simulink model "purePursuitBackward"  (R2024b)
settings: Solver=VariableStepAuto  StartTime=0.0  StopTime=4  RelTol=1e-3
PreLoadFcn:
  | setUpPurePursuitCurveLowVel
model workspace (MAT data in the model file):
  firstWarning = 0
  originalScenarioChecksum = 'F73A6DA3C723D3CA73A6F931B7A52A9C'
values from neighbouring files (symbols this model uses):
  L = 3    [setUpPurePursuit.m]    (also in setUpPurePursuitCurveLowVel.m)
  ld = 5    [setUpPurePursuit.m]    (also in setUpPurePursuitCurveLowVel.m)
  waypoints = data(:, 1:2)    [setUpPurePursuit.m]    (also in setUpPurePursuitCurveLowVel.m)
undefined symbols (not defined in the file or in its folder): psi_o, X_o, xRef, Y_o, yRef
libraries: simulink_extras x2, robotalgslib x2, vehdynlibviscommon x1, Solver_SF x1, autolibshared x1
settings Model: PacingRate=0.700000  Creator=valakshe  LastModifiedBy=kejin
settings SolverCC: AlgebraicLoopSolver=TrustRegion
settings DebuggingCC: UnconnectedInputMsg=warning  UnconnectedOutputMsg=warning  UnconnectedLineMsg=warning
settings ModelReferenceCC: EnableRefExpFcnMdlSchedulingChecks=on
settings RTWCC: GPUComputeCapability=3.5  DLArmComputeVersion=19.05

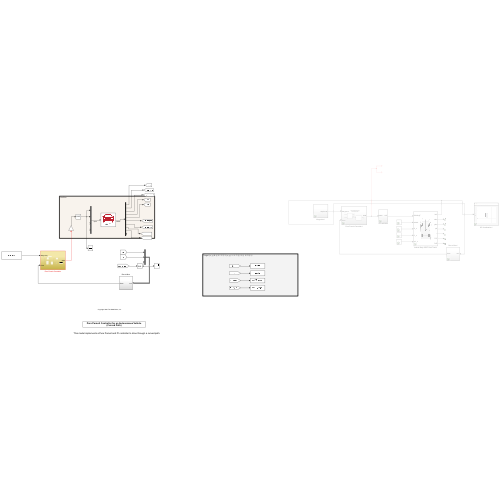
[thumbnail: Simulink's stored preview of the top-level diagram]
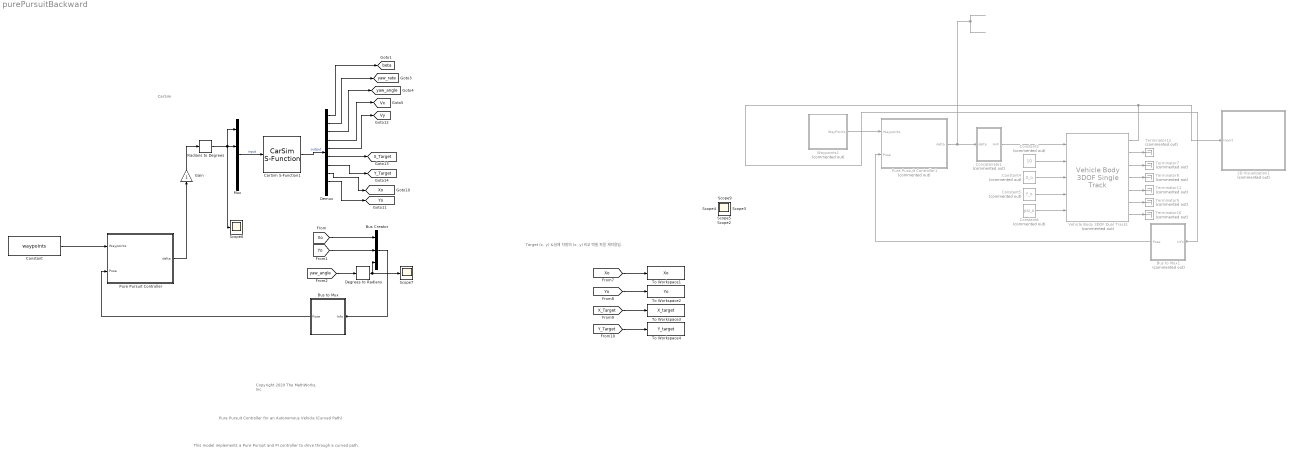
== system purePursuitBackward ==
  note: Copyright 2020 The MathWorks, Inc.
  note: Pure Pursuit Controller for an Autonomous Vehicle
      | (Curved Path)
  note: This model implements a Pure Pursuit and PI controller to drive through a curved path.
  note: CarSim
  note: Target (x, y) & 실제 차량의 (x, y) 비교 엑셀 파일 제작용임.
  2D Visualization1 : Subsystem  Commented=on
      mask Display: image("visualization.JPG");
  Bus Creator : BusCreator  Inputs=3
  Bus to Mux : Subsystem
  Bus to Mux1 : Subsystem  Commented=on
  CarSim S-Function1 : Solver_SF/CarSim S-Function  Priority=1  SIMFILE=simfile.sim  Run_RTs=off  vs_state_ind=Run  StopMode_ind=Vehicle Model
  Concatenate1 : Subsystem  Commented=on
  Constant : Constant  Value=waypoints
  Constant3 : Constant  Commented=on  Value=10
  Constant4 : Constant  Commented=on  Value=X_o
  Constant5 : Constant  Commented=on  Value=Y_o
  Constant6 : Constant  Commented=on  Value=psi_o
  Degrees to Radians : simulink_extras/Transformations/Degrees to Radians
  Demux : Demux  Outputs=10
  Gain : Gain
  Mux : Mux
  Pure Pursuit Controller : Subsystem
  Pure Pursuit Controller1 : Subsystem  Commented=on
  Radians to Degrees : simulink_extras/Transformations/Radians to Degrees
  Scope{,1..7,9} (9 alike) : Scope
  Terminator{7..12} (6 alike) : Terminator  Commented=on
  To Workspace1 : ToWorkspace  VariableName=Xo  SaveFormat=Timeseries  SampleTime=-1
  To Workspace2 : ToWorkspace  VariableName=Yo  SaveFormat=Timeseries  SampleTime=-1
  To Workspace3 : ToWorkspace  VariableName=X_target  SaveFormat=Timeseries  SampleTime=-1
  To Workspace4 : ToWorkspace  VariableName=Y_target  SaveFormat=Timeseries  SampleTime=-1
  Vehicle Body 3DOF Dual Track1 : autolibshared/Vehicle Body 3DOF Single Track  Commented=on  trackMode=Dual  inputMode=External longitudinal velocity  frontSteerMode=on  rearSteerMode=off  windMode=off  muMode=off  extFMode=off  extMMode=off  htchFMode=off  htchMMode=off  extXo=on  extpsio=on  extxdoto=off  extro=off  extYo=on  extTamb=off  extydoto=off  aMode=2  NF=2  NR=2  m=2000  a=1.4  b=1.6  h=0.35  dh=1  hh=0.2  X_o=0  xdot_o=0  CalphaMode=off  sigmaMode=on  d=0  hl=0  w=[1.4,1.4]  Cy_f=12e3  Cy_r=11e3  sigma_f=.1  sigma_r=.1  alpha_f_brk=[-.1 .1]  Cy_f_data=[-9e3 9e3]  alpha_r_brk=[-.1 .1]  Cy_r_data=[-9e3 9e3]  Y_o=0  ydot_o=0  Izz=4000  psi_o=0  r_o=0  Af=2  Cd=.3  Cl=.1  Cpm=.1  beta_w=[0:0.01:0.3]  Cs=[0:0.03:0.9]  Cym=[0:0.01:0.3]  Pabs=101325  Tair=273  g=9.81  mu=1  xdot_tol=.01  Fznom=5000  Fxtire_sat=7e4  Fytire_sat=7e4  longOff=0  latOff=0  vertOff=0  wrapAng=off
  Waypoints1 : Subsystem  Commented=on
  tag scope: Vx=global, Vy=global, X_Target=global, Xo=global, Y_Target=global, Yo=global, beta=global, yaw_angle=global, yaw_rate=global
  wires:
  Bus to Mux/1(Pose) -> Pure Pursuit Controller/2(Pose)
  Demux/3 -> [yaw_angle]
  Demux/6 -> [X_Target]
  Demux/7 -> [Y_Target]
  Demux/1 -> [beta]
  Demux/4 -> [Vx]
  Demux/5 -> [Vy]
  Mux/1 -> CarSim S-Function1/1  "input"
  CarSim S-Function1/1 -> Demux/1  "output"
  Demux/2 -> [yaw_rate]
  Demux/8 -> [Xo]
  Demux/9 -> [Yo]
  Vehicle Body 3DOF Dual Track1/5 -> Terminator11/1
  Bus to Mux1/1(Pose) -> Pure Pursuit Controller1/2(Pose)
  Vehicle Body 3DOF Dual Track1/4 -> Terminator8/1
  Vehicle Body 3DOF Dual Track1/2 -> Terminator12/1
  Constant4/1 -> Vehicle Body 3DOF Dual Track1/3
  Vehicle Body 3DOF Dual Track1/6 -> Terminator9/1
  Pure Pursuit Controller1/1(delta) -> Concatenate1/1(delta)
  Constant5/1 -> Vehicle Body 3DOF Dual Track1/4
  Constant6/1 -> Vehicle Body 3DOF Dual Track1/5
  Vehicle Body 3DOF Dual Track1/3 -> Terminator7/1
  Waypoints1/1(WayPoints) -> Pure Pursuit Controller1/1(Waypoints)
  Concatenate1/1(AnF) -> Vehicle Body 3DOF Dual Track1/1
  Vehicle Body 3DOF Dual Track1/7 -> Terminator10/1
  Vehicle Body 3DOF Dual Track1/1 -> Bus to Mux1/1(Info), 2D Visualization1/1(Inport)
  Constant3/1 -> Vehicle Body 3DOF Dual Track1/2
  Bus Creator/1 -> Bus to Mux/1(Info)
  [Xo] -> Bus Creator/1
  [Yo] -> Bus Creator/2
  [yaw_angle] -> Degrees to Radians/1
  [Y_Target] -> To Workspace4/1
  [Yo] -> To Workspace2/1
  [X_Target] -> To Workspace3/1
  [Xo] -> To Workspace1/1
  Degrees to Radians/1 -> Bus Creator/3, Scope7/1
  Radians to Degrees/1 -> Scope6/1, Mux/2, Mux/1
  Constant/1 -> Pure Pursuit Controller/1(Waypoints)
  Gain/1 -> Radians to Degrees/1
  Pure Pursuit Controller/1(delta) -> Gain/1

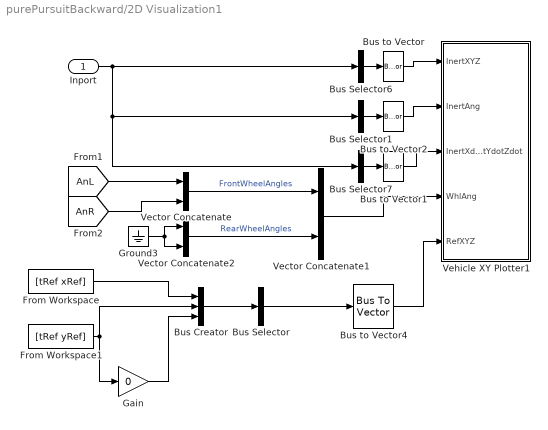
== system purePursuitBackward/2D Visualization1 ==
  Inport : Inport
  Bus Creator : BusCreator  Inputs=3
  Bus Selector : BusSelector  OutputSignals=signal1,signal2,signal3  OutputAsBus=on
  Bus Selector1 : BusSelector  OutputSignals=InertFrm.Cg.Ang.phi,InertFrm.Cg.Ang.theta,InertFrm.Cg.Ang.psi  OutputAsBus=on
  Bus Selector6 : BusSelector  OutputSignals=InertFrm.Geom.Disp.X,InertFrm.Geom.Disp.Y,InertFrm.Geom.Disp.Z  OutputAsBus=on
  Bus Selector7 : BusSelector  OutputSignals=InertFrm.Geom.Vel.Xdot,InertFrm.Geom.Vel.Ydot,InertFrm.Geom.Vel.Zdot  OutputAsBus=on
  Bus to Vector{,1..2,4} (4 alike) : BusToVector
  From Workspace : FromWorkspace  VariableName=[tRef xRef]
  From Workspace1 : FromWorkspace  VariableName=[tRef yRef]
  Gain : Gain  Gain=0
  Ground3 : Ground
  Vector Concatenate : Concatenate
  Vector Concatenate1 : Concatenate
  Vector Concatenate2 : Concatenate
  Vehicle XY Plotter1 : Subsystem  mask(Vehicle XY Plotter){extRef=on, extStats=off, extTireF=off, a=2, b=2, w=2, figBorder=10, bufferSize=1024, velNorm=5, tireFNorm=1000, pltDT=0.2}
      mask prompts: extRef "Plot path reference, extRef"; extStats "Display speed, RPM and Gear"; extTireF "Display tire forces"; a "Distance to front axle from CG, a [m]:"; b "Distance to rear axle from CG, b [m]:"; w "Track width, w [m]:"; figBorder "Distance to figure borders, figBorder [m]:"; bufferSize "Path buffer sampe size, bufferSize []:"; velNorm "Velocity vector scaling, velNorm [m*s/m]:"; tireFNorm "Tire force vector scaling, tireFNorm [m/N]:"; pltDT "Plot update rate, pltDT [s]:"
      mask help:
      | This block will display a MATLAB figure which indicates the vehicle path, current position and heading velocity.
      | An optional path reference is also provided.
      mask init:
      | block = gcb;
      | if autoblkschecksimstopped(block)
      |     ParamNames = {'extRef';'extStats';'extTireF';'extTireF'};
      |     PortNames = {'RefXYZ';'Stats';'TireFx';'TireFy'};
      |     for idx=1:length(PortNames)
      |         InportOption  = {'built-in/Ground', [PortNames{idx}, ' Ground'];...
      |             'built-in/Inport',PortNames{idx}};
      |         if ~strcmp(get_param(block,ParamNames{idx}),'on')
      |             NewBlkHdl = autoblksreplaceblock(block, InportOption, 1);
      |             set_param(NewBlkHdl, 'ShowName', 'off');
      |         else
      |             autoblksreplaceblock(block, InportOption, 2);
      |         end
      |     end
      |     InportNames = {'InertXYZ';'InertAng';'InertXdotYdotZdot';'WhlAng';'RefXYZ';'Stats';'TireFx';'TireFy'};
      |     FoundNames = get_param(find_system(block, 'LookUnderMasks', 'all', 'SearchDepth', 1, 'FollowLinks', 'on', 'BlockType', 'Inport'), 'Name');
      |     [~,PortI] = intersect(InportNames, FoundNames);
      |     PortI = sort(PortI);
      |     for idx = 1:length(PortI)
      |         set_param([block, '/', InportNames{PortI(idx)}], 'Port', num2str(idx));
      |     end
      | end
      mask TypeOptions a: Vehicle XY Plotter/a
      mask TypeOptions b: Vehicle XY Plotter/b
      mask TypeOptions w: Vehicle XY Plotter/w
      mask TypeOptions figBorder: Vehicle XY Plotter/figBorder
      mask TypeOptions bufferSize: Vehicle XY Plotter/bufferSize
      mask TypeOptions velNorm: Vehicle XY Plotter/velNorm
      mask TypeOptions tireFNorm: Vehicle XY Plotter/tireFNorm
      mask DialogControl Container3 Prompt: Plot and Display Options
  wires:
  Vector Concatenate1/1 -> Vehicle XY Plotter1/4(WhlAng)
  Ground3/1 -> Vector Concatenate2/1, Vector Concatenate2/2
  Bus Selector6/1 -> Bus to Vector/1
  Vector Concatenate/1 -> Vector Concatenate1/1  "FrontWheelAngles"
  [AnL] -> Vector Concatenate/1
  Vector Concatenate2/1 -> Vector Concatenate1/2  "RearWheelAngles"
  Bus Selector7/1 -> Bus to Vector1/1
  Bus to Vector1/1 -> Vehicle XY Plotter1/3(InertXdotYdotZdot)
  Bus to Vector/1 -> Vehicle XY Plotter1/1(InertXYZ)
  Bus to Vector2/1 -> Vehicle XY Plotter1/2(InertAng)
  Bus Selector1/1 -> Bus to Vector2/1
  [AnR] -> Vector Concatenate/2
  Inport/1 -> Bus Selector7/1, Bus Selector1/1, Bus Selector6/1
  Bus to Vector4/1 -> Vehicle XY Plotter1/5(RefXYZ)
  Bus Selector/1 -> Bus to Vector4/1
  From Workspace1/1 -> Gain/1, Bus Creator/2
  Gain/1 -> Bus Creator/3
  From Workspace/1 -> Bus Creator/1
  Bus Creator/1 -> Bus Selector/1

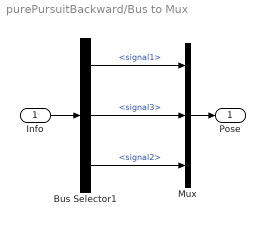
== system purePursuitBackward/Bus to Mux ==
  Info : Inport
  Bus Selector1 : BusSelector  OutputSignals=signal1,signal3,signal2
  Mux : Mux  Inputs=3
  Pose : Outport
  wires:
  Bus Selector1/3 -> Mux/3  "<signal2>"
  Bus Selector1/1 -> Mux/1  "<signal1>"
  Mux/1 -> Pose/1
  Bus Selector1/2 -> Mux/2  "<signal3>"
  Info/1 -> Bus Selector1/1

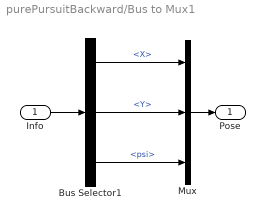
== system purePursuitBackward/Bus to Mux1 ==
  Info : Inport
  Bus Selector1 : BusSelector  OutputSignals=InertFrm.Cg.Disp.X,InertFrm.Cg.Disp.Y,InertFrm.Cg.Ang.psi
  Mux : Mux  Inputs=3
  Pose : Outport
  wires:
  Bus Selector1/3 -> Mux/3  "<psi>"
  Bus Selector1/1 -> Mux/1  "<X>"
  Mux/1 -> Pose/1
  Bus Selector1/2 -> Mux/2  "<Y>"
  Info/1 -> Bus Selector1/1

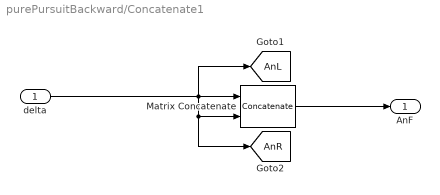
== system purePursuitBackward/Concatenate1 ==
  delta : Inport
  Matrix Concatenate : Concatenate
  AnF : Outport  VectorParamsAs1DForOutWhenUnconnected=off
  tag scope: AnL=global, AnR=global
  wires:
  Matrix Concatenate/1 -> AnF/1
  delta/1 -> [AnL], [AnR], Matrix Concatenate/2, Matrix Concatenate/1

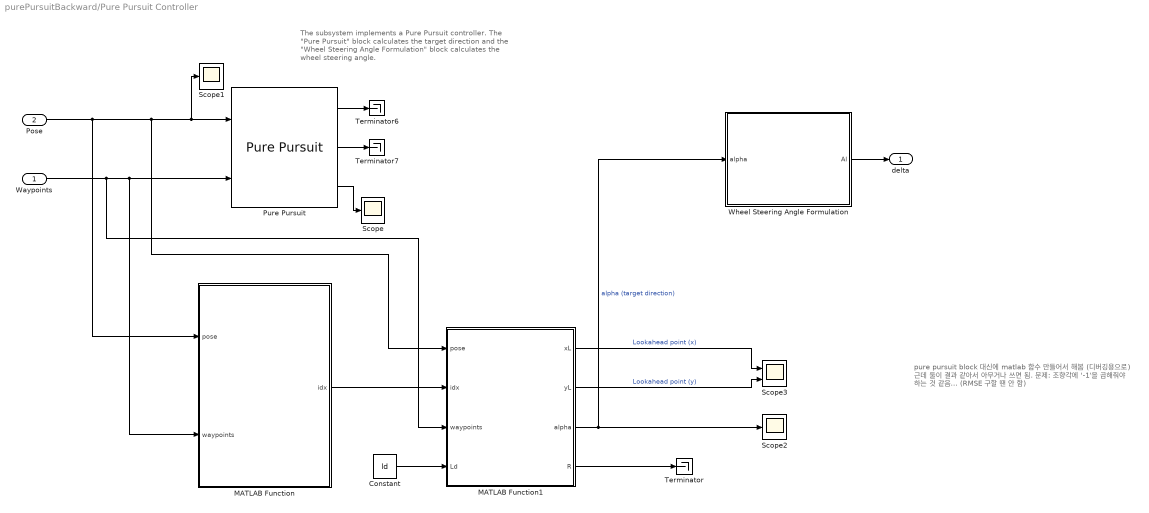
== system purePursuitBackward/Pure Pursuit Controller ==
  note: The subsystem implements a Pure Pursuit controller. The "Pure Pursuit" block calculates the target direction and the "Wheel Steering Angle Formulation" block calculates the wheel steering angle.
  note: pure pursuit block 대신에 matlab 함수 만들어서 해봄 (디버깅용으로)
      | 근데 둘이 결과 같아서 아무거나 쓰면 됨.
      | 문제: 조향각에 '-1'을 곱해줘야 하는 것 같음...
      | (RMSE 구할 땐 안 함)
  Waypoints : Inport
  Pose : Inport  Port=2
  Constant : Constant  Value=ld
  MATLAB Function : MATLAB Function  TreatAsAtomicUnit=on
  MATLAB Function1 : MATLAB Function  TreatAsAtomicUnit=on
  Pure Pursuit : robotalgslib/Pure Pursuit  DesiredLinearVelocityPort=off  DesiredLinearVelocity=0.1  MaxAngularVelocity=1.0  LookaheadDistancePort=off  LookaheadDistance=ld  TargetDirPort=on  SimulateUsing=Code generation
  Scope : Scope
  Scope1 : Scope
  Scope2 : Scope
  Scope3 : Scope  NumInputPorts=2
  Terminator : Terminator
  Terminator6 : Terminator
  Terminator7 : Terminator
  Wheel Steering Angle Formulation : Subsystem  mask{L=L, ld=ld}
      mask prompts: L "Bicycle length"; ld "Lookahead distance"
      mask TypeOptions L: Bicycle length/Value
      mask TypeOptions ld: Lookahead distance/Value
      mask Display:
      | image("GeometryMask.png")
      | port_label('input', 1, 'alpha')
      | port_label('output', 1, 'delta')
  delta : Outport
  wires:
  Wheel Steering Angle Formulation/1(Al) -> delta/1
  Pure Pursuit/3 -> Scope/1
  Waypoints/1 -> MATLAB Function1/3(waypoints), MATLAB Function/2(waypoints), Pure Pursuit/2
  Pure Pursuit/2 -> Terminator7/1
  Pose/1 -> MATLAB Function1/1(pose), Scope1/1, Pure Pursuit/1, MATLAB Function/1(pose)
  Pure Pursuit/1 -> Terminator6/1
  MATLAB Function/1(idx) -> MATLAB Function1/2(idx)
  Constant/1 -> MATLAB Function1/4(Ld)
  MATLAB Function1/3(alpha) -> Wheel Steering Angle Formulation/1(alpha), Scope2/1  "alpha (target direction)"
  MATLAB Function1/1(xL) -> Scope3/1  "Lookahead point (x)"
  MATLAB Function1/2(yL) -> Scope3/2  "Lookahead point (y)"
  MATLAB Function1/4(R) -> Terminator/1

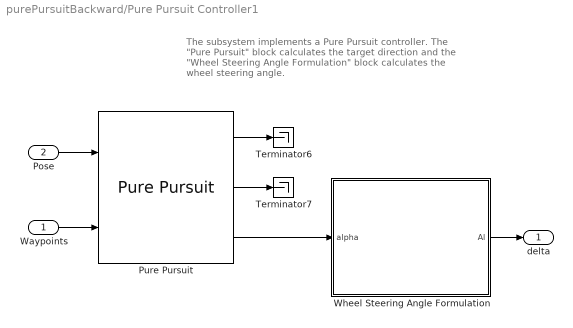
== system purePursuitBackward/Pure Pursuit Controller1 ==
  note: The subsystem implements a Pure Pursuit controller. The "Pure Pursuit" block calculates the target direction and the "Wheel Steering Angle Formulation" block calculates the wheel steering angle.
  Waypoints : Inport
  Pose : Inport  Port=2
  Pure Pursuit : robotalgslib/Pure Pursuit  DesiredLinearVelocityPort=off  DesiredLinearVelocity=0.1  MaxAngularVelocity=1.0  LookaheadDistancePort=off  LookaheadDistance=ld  TargetDirPort=on  SimulateUsing=Code generation
  Terminator6 : Terminator
  Terminator7 : Terminator
  Wheel Steering Angle Formulation : Subsystem  mask{L=L, ld=ld}
      mask prompts: L "Bicycle length"; ld "Lookahead distance"
      mask TypeOptions L: Bicycle length/Value
      mask TypeOptions ld: Lookahead distance/Value
      mask Display:
      | image("GeometryMask.png")
      | port_label('input', 1, 'alpha')
      | port_label('output', 1, 'delta')
  delta : Outport
  wires:
  Wheel Steering Angle Formulation/1(Al) -> delta/1
  Pure Pursuit/3 -> Wheel Steering Angle Formulation/1(alpha)
  Waypoints/1 -> Pure Pursuit/2
  Pure Pursuit/2 -> Terminator7/1
  Pose/1 -> Pure Pursuit/1
  Pure Pursuit/1 -> Terminator6/1

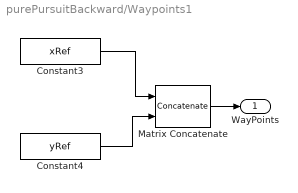
== system purePursuitBackward/Waypoints1 ==
  Constant3 : Constant  Value=xRef  SampleTime=0.1
  Constant4 : Constant  Value=yRef  SampleTime=0.1
  Matrix Concatenate : Concatenate  Mode=Multidimensional array  ConcatenateDimension=2
  WayPoints : Outport
  wires:
  Constant4/1 -> Matrix Concatenate/2
  Constant3/1 -> Matrix Concatenate/1
  Matrix Concatenate/1 -> WayPoints/1

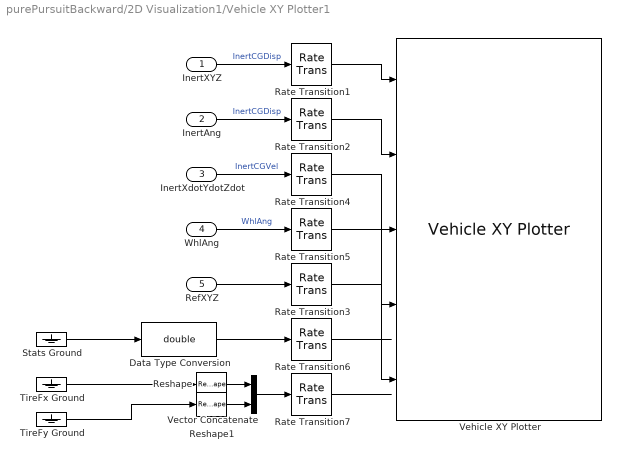
== system purePursuitBackward/2D Visualization1/Vehicle XY Plotter1 ==
  InertXYZ : Inport
  InertAng : Inport  Port=2
  InertXdotYdotZdot : Inport  Port=3
  WhlAng : Inport  Port=4
  RefXYZ : Inport  Port=5
  Data Type Conversion : DataTypeConversion  OutDataTypeStr=double  SaturateOnIntegerOverflow=off  RndMeth=Floor
  Rate Transition{1..7} (7 alike) : RateTransition  Deterministic=off  OutPortSampleTime=pltDT
  Reshape : Reshape  OutputDimensionality=Row vector (2-D)
  Reshape1 : Reshape  OutputDimensionality=Row vector (2-D)
  Stats Ground : Ground
  TireFx Ground : Ground
  TireFy Ground : Ground
  Vector Concatenate : Concatenate  Mode=Multidimensional array
  Vehicle XY Plotter : vehdynlibviscommon/Vehicle XY Plotter  w=w  a=a  b=b  figBorder=figBorder  bufferSize=bufferSize  extStats=off  extTireF=off
  wires:
  Vector Concatenate/1 -> Rate Transition7/1
  Reshape1/1 -> Vector Concatenate/2
  Reshape/1 -> Vector Concatenate/1
  RefXYZ/1 -> Rate Transition3/1
  Rate Transition7/1 -> ?
  Data Type Conversion/1 -> Rate Transition6/1
  Rate Transition6/1 -> ?
  Rate Transition5/1 -> Vehicle XY Plotter/4
  Rate Transition4/1 -> Vehicle XY Plotter/3
  Rate Transition2/1 -> Vehicle XY Plotter/2
  Rate Transition1/1 -> Vehicle XY Plotter/1
  Rate Transition3/1 -> Vehicle XY Plotter/5
  WhlAng/1 -> Rate Transition5/1  "WhlAng"
  InertXYZ/1 -> Rate Transition1/1  "InertCGDisp"
  InertXdotYdotZdot/1 -> Rate Transition4/1  "InertCGVel"
  InertAng/1 -> Rate Transition2/1  "InertCGDisp"
  TireFx Ground/1 -> Reshape/1
  TireFy Ground/1 -> Reshape1/1
  Stats Ground/1 -> Data Type Conversion/1

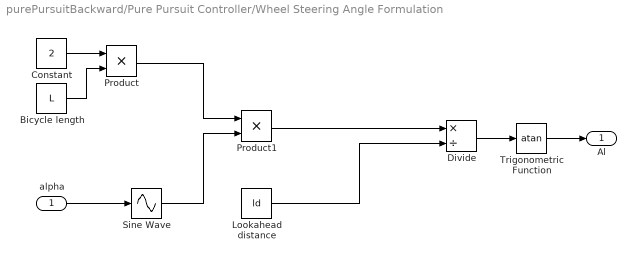
== system purePursuitBackward/Pure Pursuit Controller/Wheel Steering Angle Formulation ==
  alpha : Inport
  Bicycle length : Constant  Value=L
  Constant : Constant  Value=2
  Divide : Product  Inputs=*/
  Lookahead distance : Constant  Value=ld
  Product : Product
  Product1 : Product
  Sine Wave : Sin  TimeSource=Use external signal  SampleTime=0
  Trigonometric Function : Trigonometry  Operator=atan
  Al : Outport
  wires:
  Sine Wave/1 -> Product1/2
  Constant/1 -> Product/1
  Product1/1 -> Divide/1
  Product/1 -> Product1/1
  Divide/1 -> Trigonometric Function/1
  Trigonometric Function/1 -> Al/1
  alpha/1 -> Sine Wave/1
  Bicycle length/1 -> Product/2
  Lookahead distance/1 -> Divide/2

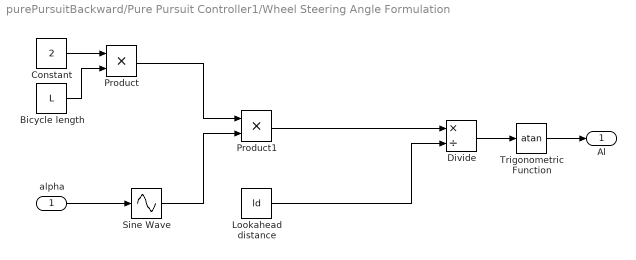
== system purePursuitBackward/Pure Pursuit Controller1/Wheel Steering Angle Formulation ==
  alpha : Inport
  Bicycle length : Constant  Value=L
  Constant : Constant  Value=2
  Divide : Product  Inputs=*/
  Lookahead distance : Constant  Value=ld
  Product : Product
  Product1 : Product
  Sine Wave : Sin  TimeSource=Use external signal  SampleTime=0
  Trigonometric Function : Trigonometry  Operator=atan
  Al : Outport
  wires:
  Sine Wave/1 -> Product1/2
  Bicycle length/1 -> Product/2
  Constant/1 -> Product/1
  Product1/1 -> Divide/1
  Product/1 -> Product1/1
  Divide/1 -> Trigonometric Function/1
  Trigonometric Function/1 -> Al/1
  alpha/1 -> Sine Wave/1
  Lookahead distance/1 -> Divide/2

== matlab function purePursuitBackward/Pure Pursuit Controller/MATLAB Function1 ==
  data: pose input; idx input; xL output; waypoints input; Ld input; yL output; alpha output; R output
% function [xL, yL] = findLookaheadPoint(idx, waypoints, Ld)
% s = 0;
% 
% for k = idx:size(waypoints,1)-1
%     p1 = waypoints(k,:);
%     p2 = waypoints(k+1,:);
%     ds = norm(p2 - p1);
% 
%     if s + ds >= Ld
%         t = (Ld - s)/ds;
%         pL = p1 + t*(p2 - p1);
%         xL = pL(1);
%         yL = pL(2);
%         return;
%     end
% 
%     s = s + ds;
% end
% 
% % 마지막 점 처리
% xL = waypoints(end,1);
% yL = waypoints(end,2);
% 
% 
% end


function [xL, yL, alpha, R] = findLookaheadPoint(pose, idx, waypoints, Ld)
if nargin < 5
    isReverse = false;   % 기본은 전진
end
% pose = [x; y; yaw]  (yaw in rad)

x   = pose(1);
y   = pose(2);
yaw = pose(3);

s = 0;

if ~isReverse
    % ===== 전진 주행: 기존과 동일 =====
    for k = idx : size(waypoints,1)-1
        p1 = waypoints(k,:);
        p2 = waypoints(k+1,:);
        ds = norm(p2 - p1);
        
        if s + ds >= Ld
            t  = (Ld - s)/ds;
            pL = p1 + t*(p2 - p1);
            xL = pL(1);
            yL = pL(2);

            dx = xL - x;
            dy = yL - y;
            R  = hypot(dx, dy);

            heading = yaw;                     % 진행 방향 = 차량 yaw
            alpha = atan2(dy, dx) - heading;
            alpha = atan2(sin(alpha), cos(alpha));  % -pi ~ pi 정규화
            return;
        end
        s = s + ds;
    end

    % Ld 만큼 못 찾으면 마지막 점 사용
    xL = waypoints(end,1);
    yL = waypoints(end,2);

else
    % ===== 후진 주행: 경로를 거꾸로 따라가며 Ld 뒤쪽을 찾음 =====
    for k = idx : -1 : 2
        p1 = waypoints(k,:);
        p2 = waypoints(k-1,:);   % 인덱스를 줄이면서 역방향으로 이동
        ds = norm(p2 - p1);
        
        if s + ds >= Ld
            t  = (Ld - s)/ds;
            % 여기도 p1 -> p2 방향으로 보간하지만,
            % k가 줄어드니 실제로는 station 이 감소하는 쪽(Ld 뒤쪽)을 찾는 것
            pL = p1 + t*(p2 - p1);
            xL = pL(1);
            yL = pL(2);

            dx = xL - x;
            dy = yL - y;
            R  = hypot(dx, dy);

            % 후진일 때 실제 진행 방향은 yaw + pi (차가 뒤로 가니까)
            heading = yaw + pi;
            alpha = atan2(dy, dx) - heading;
            alpha = atan2(sin(alpha), cos(alpha));  % -pi ~ pi
            return;
        end
        s = s + ds;
    end

    % Ld 만큼 못 찾으면 맨 처음 점 사용
    xL = waypoints(1,1);
    yL = waypoints(1,2);
end

% 공통: fallback일 때 α, R 계산
dx = xL - x;
dy = yL - y;
R  = hypot(dx, dy);

if ~isReverse
    heading = yaw;
else
    heading = yaw + pi;
end
alpha = atan2(dy, dx) - heading;
alpha = atan2(sin(alpha), cos(alpha));
end

== matlab function purePursuitBackward/Pure Pursuit Controller/MATLAB Function ==
  data: pose input; idx output; waypoints input
function idx = findNearestWaypoint(pose, waypoints)
x = pose(1); 
y = pose(2);

dx = waypoints(:,1) - x;
dy = waypoints(:,2) - y;
d  = sqrt(dx.^2 + dy.^2);

[~, idx] = min(d);
end
